simulink model "sampleModel1999"  (R2022a)
settings: Solver=FixedStepAuto  StartTime=0.0  StopTime=10.0  RelTol=1e-3
undefined symbols (not defined in the file): DiscIntNeverNeededParam, magnitude, Newton, Raphson
libraries: simulink x51, slpidlib x21
(part 1 of 3)
settings Model: SimulationMode=software-in-the-loop (sil)  Creator=lenovo  LastModifiedBy=TSMC
settings DataIOCC: InspectSignalLogs=on  SignalLoggingName=logsOut
settings OptimizationCC: DefaultParameterBehavior=Inlined  EnhancedBackFolding=on  PassReuseOutputArgsAs=Individual arguments  ZeroExternalMemoryAtStartup=off  ZeroInternalMemoryAtStartup=off  OptimizeBlockOrder=speed  DifferentSizesBufferReuse=on  OptimizationCustomize=off  EfficientTunableParamExpr=on
settings DebuggingCC: ParameterTunabilityLossMsg=error  UnconnectedInputMsg=warning  UnconnectedOutputMsg=warning  UnconnectedLineMsg=warning
settings ModelReferenceCC: UpdateModelReferenceTargets=Force
settings SFSimCC: MATLABDynamicMemAlloc=off
settings RTWCC: SystemTargetFile=ert.tlc  TemplateMakefile=ert_default_tmf  GenerateReport=on  IncludeHyperlinkInReport=on  GenerateTraceInfo=on  DLArmComputeVersion=19.05
settings CodeAppCC: ForceParamTrailComments=on  IgnoreCustomStorageClasses=off  OperatorAnnotations=on  SimulinkDataObjDesc=on  SFDataObjDesc=on  InsertBlockDesc=on
settings ERTTargetCC: TargetLangStandard=C99 (ISO)  GenerateSampleERTMain=on  SupportContinuousTime=on  InlinedParameterPlacement=NonHierarchical  ERTCustomFileTemplate=example_file_process.tlc

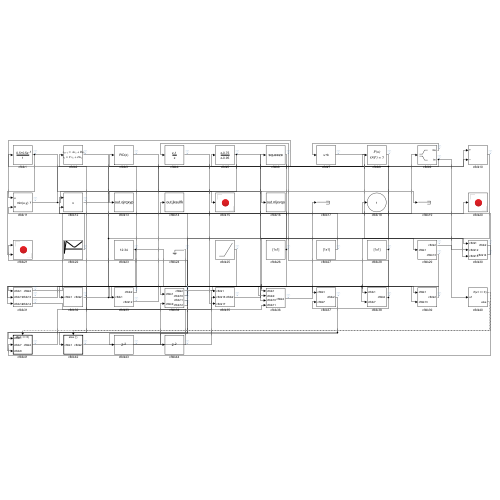
[thumbnail: Simulink's stored preview of the top-level diagram]
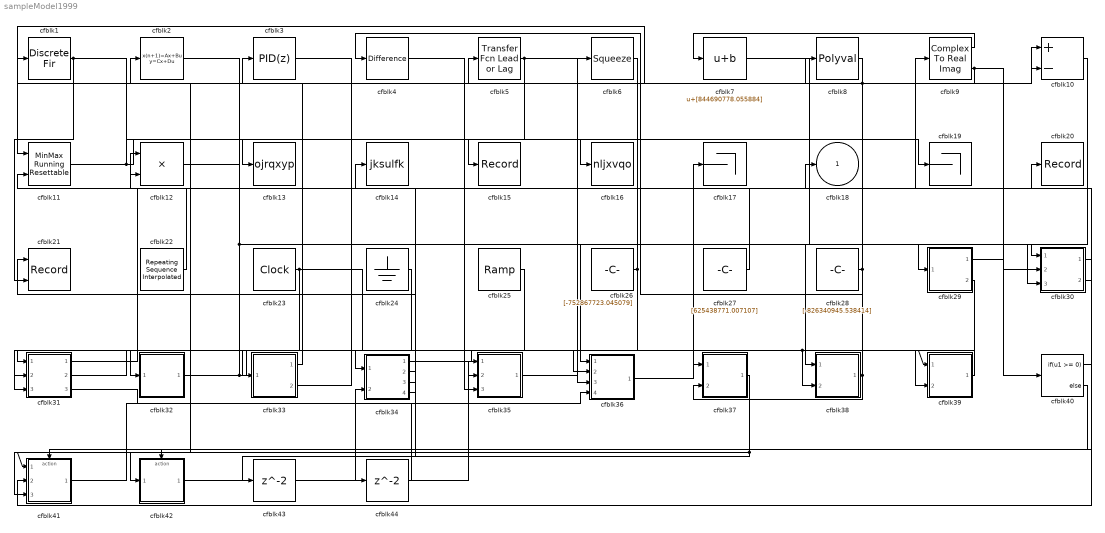
== system sampleModel1999 ==
  cfblk1 : DiscreteFir  SampleTime=1
  cfblk10 : Sum  Inputs=+-
  cfblk11 : simulink/Math Operations/MinMax Running Resettable  Function=min  vinit=0.0
  cfblk12 : Product  Inputs=**
  cfblk13 : ToWorkspace  VariableName=ojrqxyp  SaveFormat=Timeseries  SampleTime=-1
  cfblk14 : ToWorkspace  VariableName=jksulfk  SaveFormat=Timeseries  SampleTime=-1
  cfblk15 : Record  FileSettingsInternal="{\"entries\":[{\"content\":{\"excelSettings\":{\"content\":{},\"type\":\"Streamout.ExcelSettings\"}},\"type\":\"Streamout.FileSettingStorage\",\"uuid\":\"90b2dc24-f850-46d1-98e9-7d4ead9faf76\"}],\"packageUris\":[\"http://schema.mathworks.com/mf0/streamout_blocks/R2020a\"],\"version\":\"1.0\"}"  SignalsInternal="{\"entries\":[{\"content\":{\"signals\":[]},\"type\":\"RecordBlkView.InputSignals\",\"uuid\":\"4951badd-dc58-422e-9e9b-efd1dd601589\"}],\"packageUris\":[\"http://schema.mathworks.com/mf0/streamout_blocks/R2020a\"],\"version\":\"1.0\"}"  VisualizationBindings="{\"sparklinesplugin\":{\"info\":[{\"bindingParametersList\":[],\"subplotID\":1}]}}"
  cfblk16 : ToWorkspace  VariableName=nljxvqo  SaveFormat=Timeseries  SampleTime=-1
  cfblk17 : Terminator
  cfblk19 : Terminator
  cfblk2 : DiscreteStateSpace
  cfblk20 : Record  FileSettingsInternal="{\"entries\":[{\"content\":{\"excelSettings\":{\"content\":{},\"type\":\"Streamout.ExcelSettings\"}},\"type\":\"Streamout.FileSettingStorage\",\"uuid\":\"17e1182a-0793-4fff-8a02-480c6dfdb997\"}],\"packageUris\":[\"http://schema.mathworks.com/mf0/streamout_blocks/R2020a\"],\"version\":\"1.0\"}"  SignalsInternal="{\"entries\":[{\"content\":{\"signals\":[]},\"type\":\"RecordBlkView.InputSignals\",\"uuid\":\"65f435e3-1ce2-412d-96a0-f220de8eba44\"}],\"packageUris\":[\"http://schema.mathworks.com/mf0/streamout_blocks/R2020a\"],\"version\":\"1.0\"}"  VisualizationBindings="{\"sparklinesplugin\":{\"info\":[{\"bindingParametersList\":[],\"subplotID\":1}]}}"
  cfblk21 : Record  FileSettingsInternal="{\"entries\":[{\"content\":{\"excelSettings\":{\"content\":{},\"type\":\"Streamout.ExcelSettings\"}},\"type\":\"Streamout.FileSettingStorage\",\"uuid\":\"712499bb-47a7-4324-9665-446955fb75ef\"}],\"packageUris\":[\"http://schema.mathworks.com/mf0/streamout_blocks/R2020a\"],\"version\":\"1.0\"}"  Layout=[1 1]  SignalsInternal="{\"entries\":[{\"content\":{\"signals\":[]},\"type\":\"RecordBlkView.InputSignals\",\"uuid\":\"d2038af1-ceeb-4d6d-b80f-55793e10b03b\"}],\"packageUris\":[\"http://schema.mathworks.com/mf0/streamout_blocks/R2020a\"],\"version\":\"1.0\"}"  VisualizationBindings="{\"xyplotplugin\":{\"info\":[{\"series\":[],\"subplotID\":1}]}}"  CompatibilityTag=XY  st=-1
  cfblk22 : simulink/Sources/Repeating Sequence Interpolated  OutValues=[-485646331.647212, 895001609.068764, 235742497.742022, 228091536.709134, 839624606.118321]  TimeValues=[0 0.1 0.5 0.6 1].'  LookUpMeth=Use Input Below  tsamp=0.01  OutMin=[]  OutMax=[]  OutDataTypeStr=double  OutputDataTypeScalingMode=double  OutDataType=fixdt(0,8)  OutScaling=2^-10
  cfblk23 : DigitalClock
  cfblk24 : Ground
  cfblk25 : simulink/Sources/Ramp  slope=[-4406.456708]  start=[7.098891]  InitialOutput=[-211121.092474]
  cfblk26 : Constant  Value=[-752867723.045079]  SampleTime=1
  cfblk27 : Constant  Value=[625438771.007107]  SampleTime=1
  cfblk28 : Constant  Value=[-826340945.538414]  SampleTime=1
  cfblk29 : Subsystem
  cfblk3 : slpidlib/PID Controller  Controller=PID  Form=Parallel  TimeDomain=Discrete-time  UseExternalTs=off  SampleTime=1  IntegratorMethod=Forward Euler  FilterMethod=Forward Euler  ControllerParametersSource=internal  P=1  I=1  UseKiTs=off  D=0  N=100  UseFilter=on  TunerSelectOption=Transfer Function Based (PID Tuner App)  InitialConditionSource=internal  InitialConditionForIntegrator=0  InitialConditionForFilter=0  DifferentiatorICPrevScaledInput=0  ExternalReset=none  TrackingMode=off  Kt=1  LimitOutput=off  SatLimitsSource=internal  UpperSaturationLimit=inf  LowerSaturationLimit=-inf  LinearizeAsGain=off  AntiWindupMode=none  Kb=1  POutMin=[]  POutMax=[]  IOutMin=[]  IOutMax=[]  DOutMin=[]  DOutMax=[]  NOutMin=[]  NOutMax=[]  SumOutMin=[]  SumOutMax=[]  SaturationOutMin=[]  SaturationOutMax=[]  PParamMin=[]  PParamMax=[]  IParamMin=[]  IParamMax=[]  DParamMin=[]  DParamMax=[]  NParamMin=[]  NParamMax=[]  KbParamMin=[]  KbParamMax=[]  KtParamMin=[]  KtParamMax=[]  KbOutMin=[]  KbOutMax=[]  KtOutMin=[]  KtOutMax=[]  IntegratorOutMin=[]  IntegratorOutMax=[]  FilterOutMin=[]  FilterOutMax=[]  SumI1OutMin=[]  SumI1OutMax=[]  SumI2OutMin=[]  SumI2OutMax=[]  SumI3OutMin=[]  SumI3OutMax=[]  SumI4OutMin=[]  SumI4OutMax=[]  SumDOutMin=[]  SumDOutMax=[]  DifferentiatorOutMin=[]  DifferentiatorOutMax=[]  FilterDiffOutCoefMin=[]  FilterDiffOutCoefMax=[]  ReciprocalOutMin=[]  ReciprocalOutMax=[]  SumDenOutMin=[]  SumDenOutMax=[]  SumNumOutMin=[]  SumNumOutMax=[]  DivideOutMin=[]  DivideOutMax=[]  UdiffTsProdOutMin=[]  UdiffTsProdOutMax=[]  NTsProdOutMin=[]  NTsProdOutMax=[]  UintegralTsProdOutMin=[]  UintegralTsProdOutMax=[]  UngainTsProdOutMin=[]  UngainTsProdOutMax=[]  IntegratorContinuousStateAttributes=''  IntegratorStateMustResolveToSignalObject=off  IntegratorRTWStateStorageClass=Auto  FilterContinuousStateAttributes=''  FilterStateMustResolveToSignalObject=off  FilterRTWStateStorageClass=Auto  ParallelPVariant=InternalParameters  IdealPVariant=Disabled  IVariant=InternalParameters  DVariant=InternalParameters  IntegratorVariant=Discrete  SatVariant=Disabled  AWVariant=Passthrough  PCopyVariant=Disabled  TRVariant=Disabled  FdbkBlocksVariant=Forward  IdealPFdbkVariant=Disabled  SatFdbkVariant=Disabled  DerivativeFilterVariant=ForwardEulerFilter  NVariant=InternalParameters  NCopyVariant=Disabled  FilterICVariant=InternalICsFilter  IntegratorICVariant=InternalICs  ExternalResetVariant=Disabled  TRSumVariant=Passthrough  SumFdbkVariant=Disabled  SumVariant=Sum_PID  TsampFilterVariant=InternalTs  TsampNgainVariant=Passthrough  TsampIntegralVariant=Passthrough  ExternalSaturationOutDataTypeStr=Inherit: Same as second input  aMode=0
  cfblk30 : Subsystem
  cfblk31 : Subsystem
  cfblk32 : Subsystem
  cfblk33 : Subsystem
  cfblk34 : Subsystem
  cfblk35 : Subsystem
  cfblk36 : Subsystem
  cfblk37 : Subsystem
  cfblk38 : Subsystem
  cfblk39 : Subsystem
  cfblk4 : simulink/Discrete/Difference  ICPrevInput=0.0  OutMin=[]  OutMax=[]  OutDataTypeStr=Inherit: Inherit via back propagation  OutDataType=fixdt(1, 16)  OutScaling=2^-10  DoSatur=off
  cfblk40 : If  IfExpression=u1 >= 0  SampleTime=1
  cfblk41 : Subsystem  TreatAsAtomicUnit=on
  cfblk42 : Subsystem  TreatAsAtomicUnit=on
  cfblk43 : Delay  SampleTime=1
  cfblk44 : Delay  SampleTime=1
  cfblk5 : simulink/Discrete/Transfer Fcn Lead or Lag  PoleZ=0.95  ZeroZ=0.75  ICPrevOutput=0.0  ICPrevInput=0.0  DoSatur=off
      settings: SourceProductBaseCode=SL
  cfblk6 : Squeeze
  cfblk7 : Bias  Bias=[844690778.055884]  SaturateOnIntegerOverflow=off
  cfblk8 : Polyval  Coefs=[ +2.081618890e-019, -1.441693666e-014, +4.719686976e-010, -8.536869453e-006, +1.621573104e-001, -8.087801117e+001 ]
  cfblk9 : ComplexToRealImag
  cfblk18 : Outport
  wires:
  cfblk37/1(cfblk2) -> cfblk41/1(cfblk1), cfblk43/1
  cfblk6/1 -> cfblk36/1(cfblk1)
  cfblk38/1(cfblk2) -> cfblk4/1, cfblk37/2(cfblk7)
  cfblk9/1 -> cfblk7/1
  cfblk32/1(cfblk2) -> cfblk36/2(cfblk9), cfblk20/1
  cfblk8/1 -> cfblk11/1, cfblk38/1(cfblk1)
  cfblk28/1 -> cfblk1/1, cfblk31/3(cfblk12)
  cfblk3/1 -> cfblk16/1
  cfblk5/1 -> cfblk13/1, cfblk30/1(cfblk1)
  cfblk36/1(cfblk2) -> cfblk17/1
  cfblk9/2 -> cfblk5/1, cfblk30/2(cfblk12)
  cfblk33/1(cfblk2) -> cfblk3/1
  cfblk11/1 -> cfblk19/1, cfblk10/2
  cfblk7/1 -> cfblk29/1(cfblk1)
  cfblk4/1 -> cfblk36/3(cfblk10)
  cfblk1/1 -> cfblk15/1, cfblk21/2
  cfblk31/1(cfblk2) -> cfblk9/1
  cfblk30/1(cfblk2) -> cfblk41/2(cfblk7)
  cfblk25/1 -> cfblk32/1(cfblk1)
  cfblk26/1 -> cfblk12/1, cfblk31/2(cfblk11)
  cfblk22/1 -> cfblk11/2
  cfblk24/1 -> cfblk42/1(cfblk1)
  cfblk41/1(cfblk2) -> cfblk36/4(cfblk11)
  cfblk34/1(cfblk2) -> cfblk37/1(cfblk1)
  cfblk34/2(cfblk10) -> cfblk12/2
  cfblk12/1 -> cfblk10/1
  cfblk27/1 -> cfblk14/1
  cfblk2/1 -> cfblk39/1(cfblk1), cfblk38/2(cfblk7), cfblk30/3(cfblk13)
  cfblk34/3(cfblk11) -> cfblk41/3(cfblk8)
  cfblk34/4(cfblk12) -> cfblk21/1
  cfblk31/2(cfblk13) -> cfblk34/1(cfblk1)
  cfblk35/1(cfblk2) -> cfblk6/1
  cfblk42/1(cfblk2) -> cfblk35/1(cfblk1)
  cfblk30/2(cfblk14) -> cfblk18/1
  cfblk23/1 -> cfblk33/1(cfblk1), cfblk39/2(cfblk13)
  cfblk29/1(cfblk2) -> cfblk40/1
  cfblk33/2(cfblk12) -> cfblk8/1
  cfblk31/3(cfblk14) -> cfblk35/2(cfblk16)
  cfblk39/1(cfblk2) -> cfblk31/1(cfblk1)
  cfblk29/2(cfblk13) -> cfblk35/3(cfblk17)
  cfblk40/1 -> cfblk41/Action
  cfblk40/2 -> cfblk42/Action
  cfblk43/1 -> cfblk34/2(cfblk9)
  cfblk10/1 -> cfblk44/1
  cfblk44/1 -> cfblk2/1

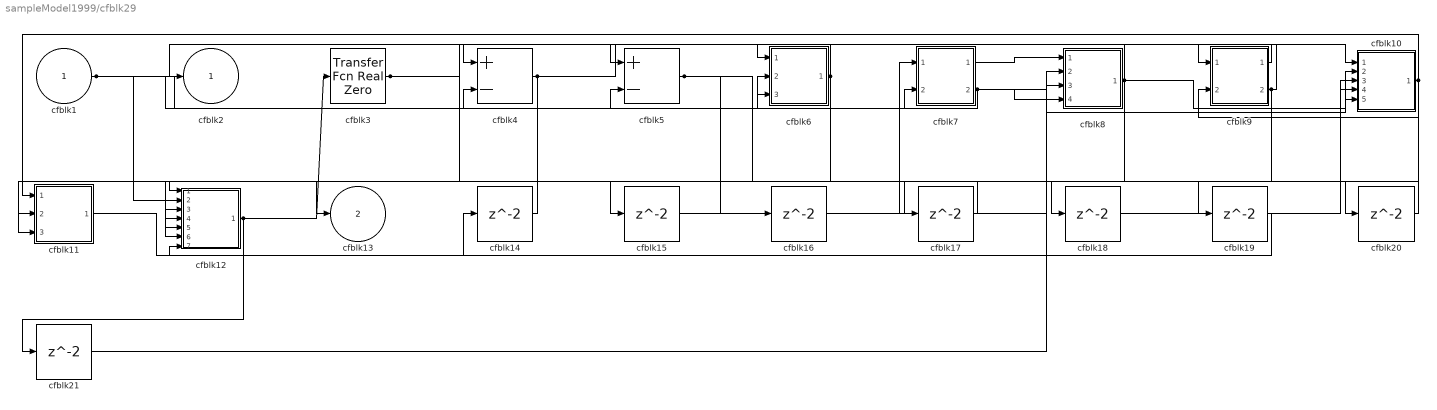
== system sampleModel1999/cfblk29 ==
  cfblk1 : Inport
  cfblk10 : Subsystem
  cfblk11 : Subsystem
  cfblk12 : Subsystem
  cfblk{14..21} (8 alike) : Delay  SampleTime=1
  cfblk3 : simulink/Discrete/Transfer Fcn Real Zero  ZeroZ=0.75  ICPrevInput=0.0  DoSatur=off
      settings: SourceProductBaseCode=SL
  cfblk4 : Sum  Inputs=+-
  cfblk5 : Sum  Inputs=+-
  cfblk6 : Subsystem
  cfblk7 : Subsystem
  cfblk8 : Subsystem
  cfblk9 : Subsystem
  cfblk2 : Outport
  cfblk13 : Outport  Port=2
  wires:
  cfblk7/1(cfblk2) -> cfblk8/1(cfblk1)
  cfblk9/1(cfblk2) -> cfblk6/1(cfblk1)
  cfblk5/1 -> cfblk16/1, cfblk17/1, cfblk18/1
  cfblk1/1 -> cfblk7/2(cfblk13), cfblk5/2, cfblk12/2(cfblk11)
  cfblk8/1(cfblk2) -> cfblk4/1, cfblk12/1(cfblk1), cfblk10/5(cfblk13)
  cfblk4/1 -> cfblk10/1(cfblk1), cfblk13/1, cfblk12/5(cfblk14), cfblk12/6(cfblk15)
  cfblk9/2(cfblk8) -> cfblk5/1, cfblk11/3(cfblk11), cfblk19/1
  cfblk12/1(cfblk2) -> cfblk3/1, cfblk21/1
  cfblk7/2(cfblk14) -> cfblk6/2(cfblk10), cfblk6/3(cfblk11), cfblk10/2(cfblk10), cfblk8/4(cfblk12)
  cfblk6/1(cfblk2) -> cfblk2/1, cfblk15/1
  cfblk3/1 -> cfblk9/1(cfblk1), cfblk20/1
  cfblk10/1(cfblk2) -> cfblk11/1(cfblk1), cfblk11/2(cfblk10), cfblk12/4(cfblk13), cfblk9/2(cfblk7)
  cfblk11/1(cfblk2) -> cfblk14/1
  cfblk14/1 -> cfblk4/2
  cfblk15/1 -> cfblk8/2(cfblk10)
  cfblk16/1 -> cfblk7/1(cfblk1)
  cfblk17/1 -> cfblk12/3(cfblk12)
  cfblk18/1 -> cfblk10/4(cfblk12)
  cfblk19/1 -> cfblk12/7(cfblk16)
  cfblk20/1 -> cfblk10/3(cfblk11)
  cfblk21/1 -> cfblk8/3(cfblk11)

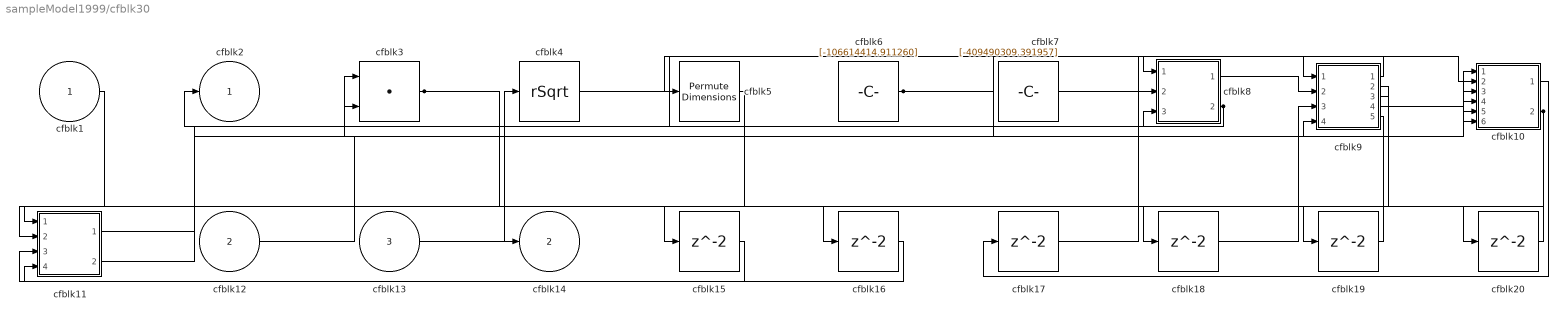
== system sampleModel1999/cfblk30 ==
  cfblk1 : Inport
  cfblk12 : Inport  Port=2
  cfblk13 : Inport  Port=3
  cfblk10 : Subsystem
  cfblk11 : Subsystem
  cfblk{15..20} (6 alike) : Delay  SampleTime=1
  cfblk3 : DotProduct  OutDataTypeStr=Inherit: Inherit via internal rule
  cfblk4 : Sqrt  Operator=rSqrt  AlgorithmType=Newton-Raphson
  cfblk5 : PermuteDimensions
  cfblk6 : Constant  Value=[-106614414.911260]  SampleTime=1
  cfblk7 : Constant  Value=[-409490309.391957]  SampleTime=1
  cfblk8 : Subsystem
  cfblk9 : Subsystem
  cfblk2 : Outport
  cfblk14 : Outport  Port=2
  wires:
  cfblk1/1 -> cfblk11/1(cfblk1)
  cfblk3/1 -> cfblk10/5(cfblk15), cfblk20/1
  cfblk11/1(cfblk2) -> cfblk8/1(cfblk1)
  cfblk12/1 -> cfblk10/1(cfblk1)
  cfblk13/1 -> cfblk4/1
  cfblk4/1 -> cfblk8/3(cfblk10)
  cfblk6/1 -> cfblk10/2(cfblk12), cfblk10/6(cfblk16)
  cfblk9/1(cfblk2) -> cfblk5/1
  cfblk7/1 -> cfblk9/1(cfblk1)
  cfblk8/1(cfblk2) -> cfblk9/2(cfblk7)
  cfblk9/2(cfblk10) -> cfblk14/1
  cfblk8/2(cfblk11) -> cfblk2/1, cfblk3/2
  cfblk9/4(cfblk12) -> cfblk10/3(cfblk13)
  cfblk11/2(cfblk15) -> cfblk10/4(cfblk14)
  cfblk10/2(cfblk17) -> cfblk18/1, cfblk19/1
  cfblk9/5(cfblk13) -> cfblk3/1
  cfblk5/1 -> cfblk15/1
  cfblk15/1 -> cfblk11/3(cfblk13)
  cfblk9/3(cfblk11) -> cfblk16/1
  cfblk16/1 -> cfblk11/4(cfblk14)
  cfblk10/1(cfblk2) -> cfblk17/1
  cfblk17/1 -> cfblk8/2(cfblk9)
  cfblk18/1 -> cfblk9/3(cfblk8)
  cfblk19/1 -> cfblk9/4(cfblk9)
  cfblk20/1 -> cfblk11/2(cfblk12)

== system sampleModel1999/cfblk31 ==
  cfblk1 : Inport
  cfblk11 : Inport  Port=2
  cfblk12 : Inport  Port=3
  cfblk10 : Subsystem
  cfblk15 : Delay  SampleTime=1
  cfblk16 : Delay  SampleTime=1
  cfblk3 : DiscreteZeroPole  Poles=[0 0.5]  Gain=1
  cfblk4 : slpidlib/PID Controller  Controller=PID  Form=Parallel  TimeDomain=Discrete-time  UseExternalTs=off  SampleTime=1  IntegratorMethod=Forward Euler  FilterMethod=Forward Euler  ControllerParametersSource=internal  P=1  I=1  UseKiTs=off  D=0  N=100  UseFilter=on  TunerSelectOption=Transfer Function Based (PID Tuner App)  InitialConditionSource=internal  InitialConditionForIntegrator=0  InitialConditionForFilter=0  DifferentiatorICPrevScaledInput=0  ExternalReset=none  TrackingMode=off  Kt=1  LimitOutput=off  SatLimitsSource=internal  UpperSaturationLimit=inf  LowerSaturationLimit=-inf  LinearizeAsGain=off  AntiWindupMode=none  Kb=1  POutMin=[]  POutMax=[]  IOutMin=[]  IOutMax=[]  DOutMin=[]  DOutMax=[]  NOutMin=[]  NOutMax=[]  SumOutMin=[]  SumOutMax=[]  SaturationOutMin=[]  SaturationOutMax=[]  PParamMin=[]  PParamMax=[]  IParamMin=[]  IParamMax=[]  DParamMin=[]  DParamMax=[]  NParamMin=[]  NParamMax=[]  KbParamMin=[]  KbParamMax=[]  KtParamMin=[]  KtParamMax=[]  KbOutMin=[]  KbOutMax=[]  KtOutMin=[]  KtOutMax=[]  IntegratorOutMin=[]  IntegratorOutMax=[]  FilterOutMin=[]  FilterOutMax=[]  SumI1OutMin=[]  SumI1OutMax=[]  SumI2OutMin=[]  SumI2OutMax=[]  SumI3OutMin=[]  SumI3OutMax=[]  SumI4OutMin=[]  SumI4OutMax=[]  SumDOutMin=[]  SumDOutMax=[]  DifferentiatorOutMin=[]  DifferentiatorOutMax=[]  FilterDiffOutCoefMin=[]  FilterDiffOutCoefMax=[]  ReciprocalOutMin=[]  ReciprocalOutMax=[]  SumDenOutMin=[]  SumDenOutMax=[]  SumNumOutMin=[]  SumNumOutMax=[]  DivideOutMin=[]  DivideOutMax=[]  UdiffTsProdOutMin=[]  UdiffTsProdOutMax=[]  NTsProdOutMin=[]  NTsProdOutMax=[]  UintegralTsProdOutMin=[]  UintegralTsProdOutMax=[]  UngainTsProdOutMin=[]  UngainTsProdOutMax=[]  IntegratorContinuousStateAttributes=''  IntegratorStateMustResolveToSignalObject=off  IntegratorRTWStateStorageClass=Auto  FilterContinuousStateAttributes=''  FilterStateMustResolveToSignalObject=off  FilterRTWStateStorageClass=Auto  ParallelPVariant=InternalParameters  IdealPVariant=Disabled  IVariant=InternalParameters  DVariant=InternalParameters  IntegratorVariant=Discrete  SatVariant=Disabled  AWVariant=Passthrough  PCopyVariant=Disabled  TRVariant=Disabled  FdbkBlocksVariant=Forward  IdealPFdbkVariant=Disabled  SatFdbkVariant=Disabled  DerivativeFilterVariant=ForwardEulerFilter  NVariant=InternalParameters  NCopyVariant=Disabled  FilterICVariant=InternalICsFilter  IntegratorICVariant=InternalICs  ExternalResetVariant=Disabled  TRSumVariant=Passthrough  SumFdbkVariant=Disabled  SumVariant=Sum_PID  TsampFilterVariant=InternalTs  TsampNgainVariant=Passthrough  TsampIntegralVariant=Passthrough  ExternalSaturationOutDataTypeStr=Inherit: Same as second input  aMode=0
  cfblk5 : Abs  SaturateOnIntegerOverflow=off
  cfblk6 : Constant  Value=[386910911.737461]  SampleTime=1
  cfblk7 : Subsystem
  cfblk8 : Subsystem
  cfblk9 : Subsystem
  cfblk2 : Outport
  cfblk13 : Outport  Port=2
  cfblk14 : Outport  Port=3
  wires:
  cfblk3/1 -> cfblk2/1
  cfblk6/1 -> cfblk8/2(cfblk8), cfblk9/4(cfblk9)
  cfblk10/1(cfblk2) -> cfblk3/1
  cfblk12/1 -> cfblk13/1
  cfblk9/1(cfblk2) -> cfblk7/1(cfblk1)
  cfblk10/2(cfblk15) -> cfblk7/2(cfblk8)
  cfblk4/1 -> cfblk10/1(cfblk1), cfblk9/2(cfblk7), cfblk9/5(cfblk10)
  cfblk1/1 -> cfblk8/3(cfblk9)
  cfblk8/1(cfblk2) -> cfblk5/1
  cfblk11/1 -> cfblk10/2(cfblk14), cfblk9/3(cfblk8), cfblk7/3(cfblk9), cfblk7/4(cfblk10)
  cfblk5/1 -> cfblk9/1(cfblk1)
  cfblk7/2(cfblk11) -> cfblk14/1
  cfblk7/1(cfblk2) -> cfblk15/1
  cfblk15/1 -> cfblk8/1(cfblk1)
  cfblk10/3(cfblk16) -> cfblk16/1
  cfblk16/1 -> cfblk4/1

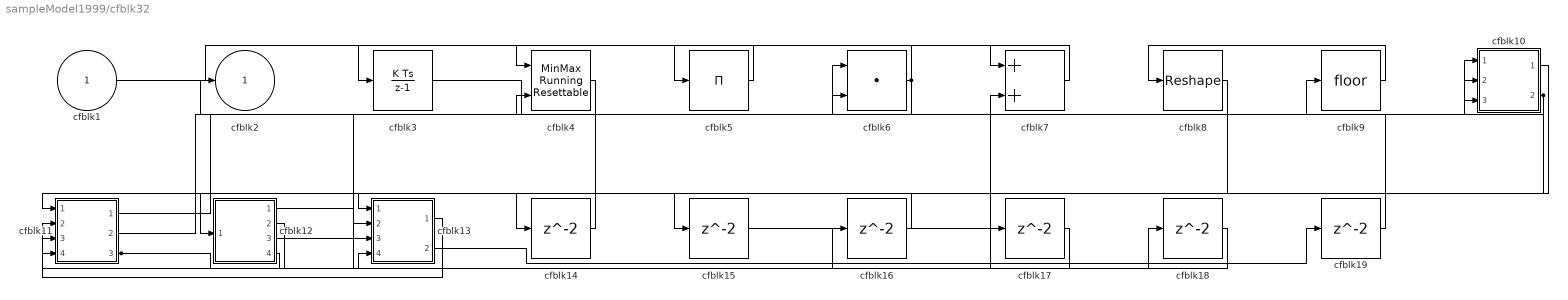
== system sampleModel1999/cfblk32 ==
  cfblk1 : Inport
  cfblk10 : Subsystem
  cfblk11 : Subsystem
  cfblk12 : Subsystem
  cfblk13 : Subsystem
  cfblk{14..19} (6 alike) : Delay  SampleTime=1
  cfblk3 : DiscreteIntegrator  ICPrevOutput=DiscIntNeverNeededParam  ICPrevScaledInput=DiscIntNeverNeededParam
  cfblk4 : simulink/Math Operations/MinMax Running Resettable  Function=min  vinit=0.0
  cfblk5 : Product  Inputs=*
  cfblk6 : DotProduct  OutDataTypeStr=Inherit: Inherit via internal rule
  cfblk7 : Sum
  cfblk8 : Reshape
  cfblk9 : Rounding
  cfblk2 : Outport
  wires:
  cfblk11/1(cfblk2) -> cfblk10/1(cfblk1)
  cfblk8/1 -> cfblk12/1(cfblk1)
  cfblk7/1 -> cfblk5/1
  cfblk5/1 -> cfblk3/1
  cfblk9/1 -> cfblk8/1
  cfblk1/1 -> cfblk7/1
  cfblk4/1 -> cfblk13/1(cfblk1)
  cfblk6/1 -> cfblk4/1, cfblk4/2
  cfblk12/1(cfblk2) -> cfblk6/1
  cfblk10/2(cfblk12) -> cfblk2/1, cfblk15/1
  cfblk11/2(cfblk12) -> cfblk10/2(cfblk10)
  cfblk11/3(cfblk13) -> cfblk16/1, cfblk17/1, cfblk18/1
  cfblk13/1(cfblk2) -> cfblk11/2(cfblk9)
  cfblk12/2(cfblk13) -> cfblk11/3(cfblk10)
  cfblk3/1 -> cfblk9/1
  cfblk12/3(cfblk14) -> cfblk10/3(cfblk11)
  cfblk12/4(cfblk15) -> cfblk11/4(cfblk11)
  cfblk10/1(cfblk2) -> cfblk14/1
  cfblk14/1 -> cfblk11/1(cfblk1)
  cfblk15/1 -> cfblk7/2
  cfblk16/1 -> cfblk13/2(cfblk8)
  cfblk17/1 -> cfblk13/3(cfblk9)
  cfblk18/1 -> cfblk13/4(cfblk10)
  cfblk13/2(cfblk11) -> cfblk19/1
  cfblk19/1 -> cfblk6/2

== system sampleModel1999/cfblk33 ==
  cfblk1 : Inport
  cfblk10 : Subsystem
  cfblk11 : Subsystem
  cfblk13 : Delay  SampleTime=1
  cfblk14 : Delay  SampleTime=1
  cfblk3 : DiscreteTransferFcn  SampleTime=1
  cfblk4 : PermuteDimensions
  cfblk5 : Product  Inputs=*
  cfblk6 : Abs  SaturateOnIntegerOverflow=off
  cfblk7 : Constant  Value=[-887141361.180652]  SampleTime=1
  cfblk8 : Subsystem
  cfblk9 : Subsystem
  cfblk2 : Outport
  cfblk12 : Outport  Port=2
  wires:
  cfblk3/1 -> cfblk5/1, cfblk10/3(cfblk14), cfblk10/4(cfblk15)
  cfblk7/1 -> cfblk2/1
  cfblk4/1 -> cfblk3/1, cfblk12/1
  cfblk1/1 -> cfblk11/1(cfblk1), cfblk11/2(cfblk12)
  cfblk5/1 -> cfblk8/2(cfblk14)
  cfblk6/1 -> cfblk8/3(cfblk15), cfblk10/2(cfblk13)
  cfblk9/1(cfblk2) -> cfblk4/1
  cfblk8/1(cfblk2) -> cfblk10/1(cfblk1)
  cfblk11/1(cfblk2) -> cfblk9/1(cfblk1)
  cfblk9/2(cfblk17) -> cfblk6/1
  cfblk10/1(cfblk2) -> cfblk13/1
  cfblk13/1 -> cfblk8/1(cfblk1)
  cfblk8/2(cfblk16) -> cfblk14/1
  cfblk14/1 -> cfblk9/2(cfblk16)

== system sampleModel1999/cfblk34 ==
  cfblk1 : Inport
  cfblk9 : Inport  Port=2
  cfblk3 : Bias  Bias=[203948966.941377]  SaturateOnIntegerOverflow=off
  cfblk4 : Trigonometry
  cfblk5 : Sqrt
  cfblk6 : Assignment  DiagnosticForDimensions=Warning  IndexOptions=Index vector (dialog)  Indices=1  OutputSizes=1
  cfblk7 : Subsystem
  cfblk8 : Subsystem
  cfblk2 : Outport
  cfblk10 : Outport  Port=2
  cfblk11 : Outport  Port=3
  cfblk12 : Outport  Port=4
  wires:
  cfblk9/1 -> cfblk6/1
  cfblk5/1 -> cfblk4/1
  cfblk7/1(cfblk2) -> cfblk6/2
  cfblk7/2(cfblk9) -> cfblk3/1
  cfblk3/1 -> cfblk10/1, cfblk5/1
  cfblk8/1(cfblk2) -> cfblk12/1
  cfblk1/1 -> cfblk7/1(cfblk1), cfblk8/2(cfblk7), cfblk7/2(cfblk7), cfblk7/3(cfblk8)
  cfblk4/1 -> cfblk8/1(cfblk1)
  cfblk6/1 -> cfblk2/1
  cfblk8/2(cfblk8) -> cfblk11/1

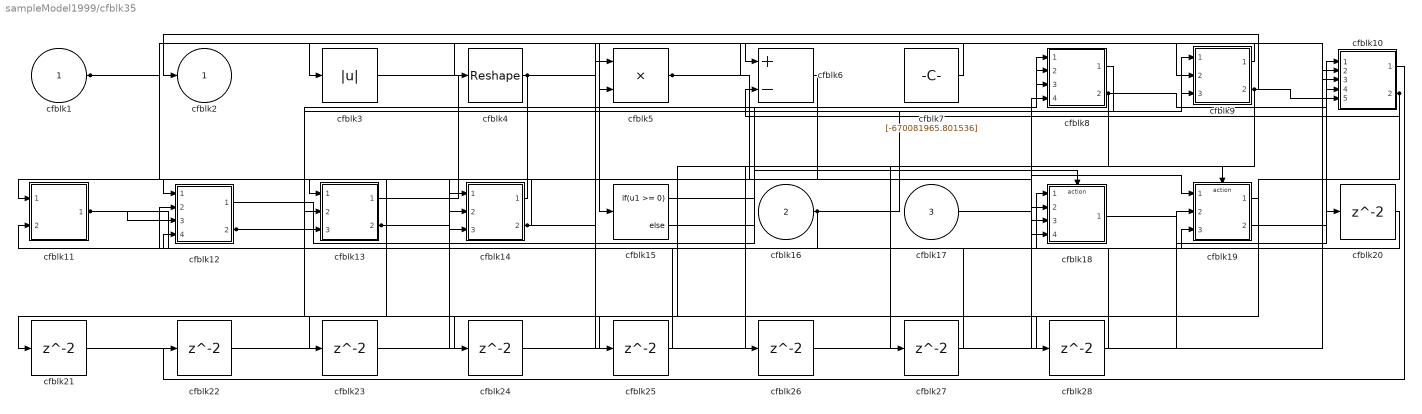
== system sampleModel1999/cfblk35 ==
  cfblk1 : Inport
  cfblk16 : Inport  Port=2
  cfblk17 : Inport  Port=3
  cfblk10 : Subsystem
  cfblk11 : Subsystem
  cfblk12 : Subsystem
  cfblk13 : Subsystem
  cfblk14 : Subsystem
  cfblk15 : If  IfExpression=u1 >= 0  SampleTime=1
  cfblk18 : Subsystem  TreatAsAtomicUnit=on
  cfblk19 : Subsystem  TreatAsAtomicUnit=on
  cfblk{20..28} (9 alike) : Delay  SampleTime=1
  cfblk3 : Abs  SaturateOnIntegerOverflow=off
  cfblk4 : Reshape
  cfblk5 : Product  Inputs=**
  cfblk6 : Sum  Inputs=+-
  cfblk7 : Constant  Value=[-670081965.801536]  SampleTime=1
  cfblk8 : Subsystem
  cfblk9 : Subsystem
  cfblk2 : Outport
  wires:
  cfblk16/1 -> cfblk9/1(cfblk1), cfblk11/2(cfblk13)
  cfblk9/1(cfblk2) -> cfblk15/1
  cfblk9/2(cfblk17) -> cfblk2/1, cfblk10/5(cfblk14), cfblk25/1, cfblk26/1
  cfblk12/1(cfblk2) -> cfblk8/1(cfblk1)
  cfblk11/1(cfblk2) -> cfblk18/1(cfblk1), cfblk12/3(cfblk15)
  cfblk5/1 -> cfblk18/2(cfblk15), cfblk9/2(cfblk15)
  cfblk13/1(cfblk2) -> cfblk18/3(cfblk16)
  cfblk3/1 -> cfblk18/4(cfblk17)
  cfblk14/1(cfblk2) -> cfblk13/1(cfblk1)
  cfblk12/2(cfblk17) -> cfblk9/3(cfblk16), cfblk8/3(cfblk12), cfblk28/1
  cfblk4/1 -> cfblk6/1, cfblk13/3(cfblk11)
  cfblk10/2(cfblk15) -> cfblk6/2, cfblk24/1
  cfblk1/1 -> cfblk14/3(cfblk15), cfblk3/1, cfblk10/3(cfblk12)
  cfblk13/2(cfblk12) -> cfblk12/1(cfblk1), cfblk19/3(cfblk12)
  cfblk17/1 -> cfblk19/1(cfblk1)
  cfblk7/1 -> cfblk4/1
  cfblk14/2(cfblk16) -> cfblk11/1(cfblk1), cfblk8/2(cfblk11)
  cfblk19/2(cfblk13) -> cfblk10/1(cfblk1)
  cfblk8/1(cfblk2) -> cfblk5/2
  cfblk8/2(cfblk14) -> cfblk10/4(cfblk13), cfblk27/1
  cfblk15/1 -> cfblk18/Action
  cfblk15/2 -> cfblk19/Action
  cfblk18/1(cfblk2) -> cfblk20/1
  cfblk20/1 -> cfblk13/2(cfblk10)
  cfblk19/1(cfblk2) -> cfblk21/1
  cfblk21/1 -> cfblk14/1(cfblk1)
  cfblk10/1(cfblk2) -> cfblk22/1
  cfblk22/1 -> cfblk5/1
  cfblk6/1 -> cfblk23/1
  cfblk23/1 -> cfblk10/2(cfblk11)
  cfblk24/1 -> cfblk19/2(cfblk11)
  cfblk25/1 -> cfblk12/4(cfblk16)
  cfblk26/1 -> cfblk8/4(cfblk13)
  cfblk27/1 -> cfblk12/2(cfblk14)
  cfblk28/1 -> cfblk14/2(cfblk14)

== system sampleModel1999/cfblk36 ==
  cfblk1 : Inport
  cfblk9 : Inport  Port=2
  cfblk10 : Inport  Port=3
  cfblk11 : Inport  Port=4
  cfblk{12..15} (4 alike) : Delay  SampleTime=1
  cfblk3 : DiscreteIntegrator  ICPrevOutput=DiscIntNeverNeededParam  ICPrevScaledInput=DiscIntNeverNeededParam
  cfblk4 : Sum  Inputs=+
  cfblk5 : Math  Operator=pow
  cfblk6 : Subsystem
  cfblk7 : Subsystem
  cfblk8 : Subsystem
  cfblk2 : Outport
  wires:
  cfblk3/1 -> cfblk6/1(cfblk1), cfblk8/4(cfblk7)
  cfblk11/1 -> cfblk4/1
  cfblk10/1 -> cfblk6/2(cfblk12), cfblk8/5(cfblk8), cfblk7/5(cfblk12)
  cfblk5/1 -> cfblk13/1, cfblk14/1, cfblk15/1
  cfblk7/1(cfblk2) -> cfblk6/4(cfblk14)
  cfblk7/2(cfblk14) -> cfblk8/1(cfblk1)
  cfblk9/1 -> cfblk7/1(cfblk1)
  cfblk1/1 -> cfblk7/3(cfblk10), cfblk6/5(cfblk15)
  cfblk4/1 -> cfblk3/1, cfblk7/4(cfblk11), cfblk5/2
  cfblk8/2(cfblk9) -> cfblk5/1
  cfblk6/1(cfblk2) -> cfblk8/2(cfblk5)
  cfblk6/2(cfblk16) -> cfblk2/1
  cfblk8/1(cfblk2) -> cfblk12/1
  cfblk12/1 -> cfblk7/2(cfblk9)
  cfblk13/1 -> cfblk6/3(cfblk13)
  cfblk14/1 -> cfblk8/3(cfblk6)
  cfblk15/1 -> cfblk7/6(cfblk13)

== system sampleModel1999/cfblk37 ==
  cfblk1 : Inport
  cfblk7 : Inport  Port=2
  cfblk10 : Delay  SampleTime=1
  cfblk3 : Sum  Inputs=+
  cfblk4 : simulink/Math Operations/MinMax Running Resettable  Function=min  vinit=0.0
  cfblk5 : ComplexToRealImag
  cfblk6 : If  IfExpression=u1 >= 0  SampleTime=1
  cfblk8 : Subsystem  TreatAsAtomicUnit=on
  cfblk9 : Subsystem  TreatAsAtomicUnit=on
  cfblk2 : Outport
  wires:
  cfblk1/1 -> cfblk2/1, cfblk4/2
  cfblk7/1 -> cfblk3/1, cfblk8/4(cfblk8)
  cfblk4/1 -> cfblk9/1(cfblk1), cfblk6/1, cfblk5/1
  cfblk9/1(cfblk2) -> cfblk8/1(cfblk1), cfblk8/5(cfblk9)
  cfblk3/1 -> cfblk9/2(cfblk13), cfblk9/4(cfblk15)
  cfblk5/1 -> cfblk8/2(cfblk6)
  cfblk5/2 -> cfblk9/3(cfblk14), cfblk8/3(cfblk7)
  cfblk6/1 -> cfblk8/Action
  cfblk6/2 -> cfblk9/Action
  cfblk8/1(cfblk2) -> cfblk10/1
  cfblk10/1 -> cfblk4/1

== system sampleModel1999/cfblk38 ==
  cfblk1 : Inport
  cfblk7 : Inport  Port=2
  cfblk3 : Sqrt  Operator=rSqrt  AlgorithmType=Newton-Raphson
  cfblk4 : ComplexToRealImag
  cfblk5 : Subsystem
  cfblk6 : Subsystem
  cfblk8 : Delay  SampleTime=1
  cfblk2 : Outport
  wires:
  cfblk1/1 -> cfblk6/2(cfblk9)
  cfblk6/1(cfblk2) -> cfblk4/1, cfblk5/2(cfblk10)
  cfblk3/1 -> cfblk6/3(cfblk10)
  cfblk7/1 -> cfblk3/1
  cfblk4/1 -> cfblk2/1
  cfblk4/2 -> cfblk5/1(cfblk1)
  cfblk5/1(cfblk2) -> cfblk8/1
  cfblk8/1 -> cfblk6/1(cfblk1)

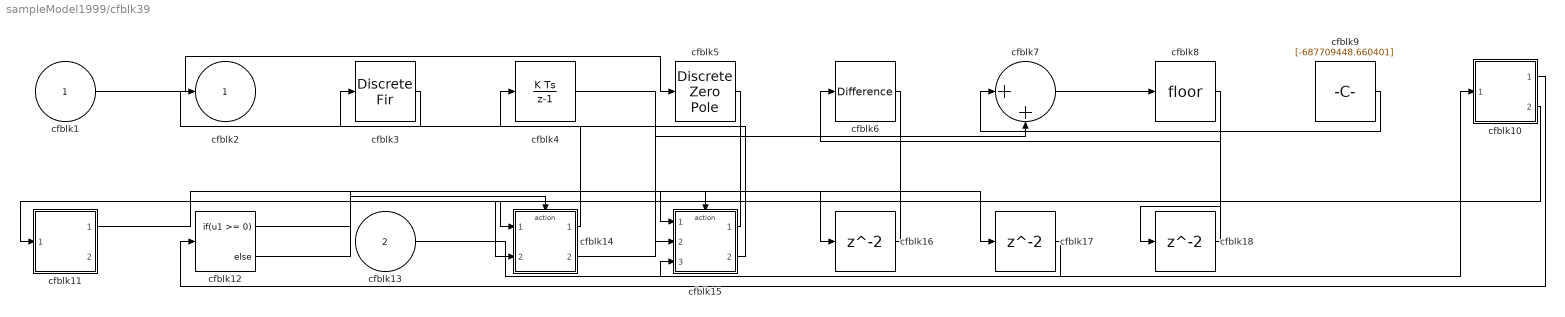
== system sampleModel1999/cfblk39 ==
  cfblk1 : Inport
  cfblk13 : Inport  Port=2
  cfblk10 : Subsystem
  cfblk11 : Subsystem
  cfblk12 : If  IfExpression=u1 >= 0  SampleTime=1
  cfblk14 : Subsystem  TreatAsAtomicUnit=on
  cfblk15 : Subsystem  TreatAsAtomicUnit=on
  cfblk16 : Delay  SampleTime=1
  cfblk17 : Delay  SampleTime=1
  cfblk18 : Delay  SampleTime=1
  cfblk3 : DiscreteFir  SampleTime=1
  cfblk4 : DiscreteIntegrator  ICPrevOutput=DiscIntNeverNeededParam  ICPrevScaledInput=DiscIntNeverNeededParam
  cfblk5 : DiscreteZeroPole  Poles=[0 0.5]  Gain=1
  cfblk6 : simulink/Discrete/Difference  ICPrevInput=0.0  OutMin=[]  OutMax=[]  OutDataTypeStr=Inherit: Inherit via back propagation  OutDataType=fixdt(1, 16)  OutScaling=2^-10  DoSatur=off
  cfblk7 : Sum  Inputs=|++
  cfblk8 : Rounding
  cfblk9 : Constant  Value=[-687709448.660401]  SampleTime=1
  cfblk2 : Outport
  wires:
  cfblk15/1(cfblk2) -> cfblk11/1(cfblk1)
  cfblk13/1 -> cfblk10/1(cfblk1)
  cfblk7/1 -> cfblk8/1
  cfblk1/1 -> cfblk5/1
  cfblk3/1 -> cfblk2/1
  cfblk5/1 -> cfblk15/2(cfblk12)
  cfblk10/1(cfblk2) -> cfblk12/1
  cfblk6/1 -> cfblk14/1(cfblk1)
  cfblk9/1 -> cfblk7/1
  cfblk15/2(cfblk14) -> cfblk4/1
  cfblk10/2(cfblk8) -> cfblk14/2(cfblk7)
  cfblk14/1(cfblk2) -> cfblk3/1
  cfblk14/2(cfblk8) -> cfblk7/2
  cfblk12/1 -> cfblk14/Action
  cfblk12/2 -> cfblk15/Action
  cfblk11/1(cfblk2) -> cfblk16/1
  cfblk16/1 -> cfblk15/1(cfblk1)
  cfblk4/1 -> cfblk17/1
  cfblk17/1 -> cfblk15/3(cfblk13)
  cfblk8/1 -> cfblk18/1
  cfblk18/1 -> cfblk6/1

== system sampleModel1999/cfblk41 ==
  cfblk1 : Inport
  cfblk7 : Inport  Port=2
  cfblk8 : Inport  Port=3
  Action Port : ActionPort  ActionPortLabel=if(u1 >= 0)
  cfblk3 : simulink/Discrete/Transfer Fcn Real Zero  ZeroZ=0.75  ICPrevInput=0.0  DoSatur=off
      settings: SourceProductBaseCode=SL
  cfblk4 : Sum  Inputs=|++
  cfblk5 : Trigonometry
  cfblk6 : Subsystem
  cfblk9 : Delay
  cfblk2 : Outport
  wires:
  cfblk8/1 -> cfblk6/1(cfblk1), cfblk6/4(cfblk7)
  cfblk5/1 -> cfblk4/1, cfblk6/3(cfblk6)
  cfblk3/1 -> cfblk5/1
  cfblk7/1 -> cfblk2/1
  cfblk1/1 -> cfblk3/1
  cfblk4/1 -> cfblk6/2(cfblk5)
  cfblk6/1(cfblk2) -> cfblk9/1
  cfblk9/1 -> cfblk4/2

== system sampleModel1999/cfblk42 ==
  cfblk1 : Inport
  Action Port : ActionPort  ActionPortLabel=else
  cfblk3 : slpidlib/PID Controller  Controller=PID  Form=Parallel  TimeDomain=Discrete-time  UseExternalTs=off  SampleTime=-1  IntegratorMethod=Forward Euler  FilterMethod=Forward Euler  ControllerParametersSource=internal  P=1  I=1  UseKiTs=off  D=0  N=100  UseFilter=on  TunerSelectOption=Transfer Function Based (PID Tuner App)  InitialConditionSource=internal  InitialConditionForIntegrator=0  InitialConditionForFilter=0  DifferentiatorICPrevScaledInput=0  ExternalReset=none  TrackingMode=off  Kt=1  LimitOutput=off  SatLimitsSource=internal  UpperSaturationLimit=inf  LowerSaturationLimit=-inf  LinearizeAsGain=off  AntiWindupMode=none  Kb=1  POutMin=[]  POutMax=[]  IOutMin=[]  IOutMax=[]  DOutMin=[]  DOutMax=[]  NOutMin=[]  NOutMax=[]  SumOutMin=[]  SumOutMax=[]  SaturationOutMin=[]  SaturationOutMax=[]  PParamMin=[]  PParamMax=[]  IParamMin=[]  IParamMax=[]  DParamMin=[]  DParamMax=[]  NParamMin=[]  NParamMax=[]  KbParamMin=[]  KbParamMax=[]  KtParamMin=[]  KtParamMax=[]  KbOutMin=[]  KbOutMax=[]  KtOutMin=[]  KtOutMax=[]  IntegratorOutMin=[]  IntegratorOutMax=[]  FilterOutMin=[]  FilterOutMax=[]  SumI1OutMin=[]  SumI1OutMax=[]  SumI2OutMin=[]  SumI2OutMax=[]  SumI3OutMin=[]  SumI3OutMax=[]  SumI4OutMin=[]  SumI4OutMax=[]  SumDOutMin=[]  SumDOutMax=[]  DifferentiatorOutMin=[]  DifferentiatorOutMax=[]  FilterDiffOutCoefMin=[]  FilterDiffOutCoefMax=[]  ReciprocalOutMin=[]  ReciprocalOutMax=[]  SumDenOutMin=[]  SumDenOutMax=[]  SumNumOutMin=[]  SumNumOutMax=[]  DivideOutMin=[]  DivideOutMax=[]  UdiffTsProdOutMin=[]  UdiffTsProdOutMax=[]  NTsProdOutMin=[]  NTsProdOutMax=[]  UintegralTsProdOutMin=[]  UintegralTsProdOutMax=[]  UngainTsProdOutMin=[]  UngainTsProdOutMax=[]  IntegratorContinuousStateAttributes=''  IntegratorStateMustResolveToSignalObject=off  IntegratorRTWStateStorageClass=Auto  FilterContinuousStateAttributes=''  FilterStateMustResolveToSignalObject=off  FilterRTWStateStorageClass=Auto  ParallelPVariant=InternalParameters  IdealPVariant=Disabled  IVariant=InternalParameters  DVariant=InternalParameters  IntegratorVariant=Discrete  SatVariant=Disabled  AWVariant=Passthrough  PCopyVariant=Disabled  TRVariant=Disabled  FdbkBlocksVariant=Forward  IdealPFdbkVariant=Disabled  SatFdbkVariant=Disabled  DerivativeFilterVariant=ForwardEulerFilter  NVariant=InternalParameters  NCopyVariant=Disabled  FilterICVariant=InternalICsFilter  IntegratorICVariant=InternalICs  ExternalResetVariant=Disabled  TRSumVariant=Passthrough  SumFdbkVariant=Disabled  SumVariant=Sum_PID  TsampFilterVariant=InternalTs  TsampNgainVariant=Passthrough  TsampIntegralVariant=Passthrough  ExternalSaturationOutDataTypeStr=Inherit: Same as second input  aMode=0
  cfblk4 : DiscreteStateSpace  SampleTime=-1
  cfblk5 : Gain  Gain=[220768961.403727]
  cfblk6 : Constant  Value=[-135023864.093883]  SampleTime=1
  cfblk7 : Subsystem
  cfblk2 : Outport
  wires:
  cfblk6/1 -> cfblk5/1
  cfblk7/1(cfblk2) -> cfblk3/1
  cfblk5/1 -> cfblk7/1(cfblk1)
  cfblk7/2(cfblk15) -> cfblk4/1
  cfblk3/1 -> cfblk2/1

== system sampleModel1999/cfblk29/cfblk10 ==
  cfblk1 : Inport
  cfblk10 : Inport  Port=2
  cfblk11 : Inport  Port=3
  cfblk12 : Inport  Port=4
  cfblk13 : Inport  Port=5
  cfblk14 : Delay  SampleTime=1
  cfblk3 : simulink/Discrete/Transfer Fcn Lead or Lag  PoleZ=0.95  ZeroZ=0.75  ICPrevOutput=0.0  ICPrevInput=0.0  DoSatur=off
      settings: SourceProductBaseCode=SL
  cfblk4 : Reshape
  cfblk5 : Sum  Inputs=+-
  cfblk6 : Squeeze
  cfblk7 : Abs  SaturateOnIntegerOverflow=off
  cfblk8 : Constant  Value=[17011813.988466]  SampleTime=1
  cfblk9 : Constant  Value=[394036538.963661]  SampleTime=1
  cfblk2 : Outport
  wires:
  cfblk9/1 -> cfblk2/1
  cfblk11/1 -> cfblk3/1
  cfblk10/1 -> cfblk5/1
  cfblk1/1 -> cfblk5/2
  cfblk12/1 -> cfblk4/1
  cfblk6/1 -> cfblk7/1
  cfblk7/1 -> cfblk14/1
  cfblk14/1 -> cfblk6/1

== system sampleModel1999/cfblk29/cfblk11 ==
  cfblk1 : Inport
  cfblk10 : Inport  Port=2
  cfblk11 : Inport  Port=3
  cfblk3 : UnitDelay  HasFrameUpgradeWarning=on
  cfblk4 : simulink/Discrete/Transfer Fcn First Order  PoleZ=0.95  ICPrevOutput=0.0  DoSatur=off
  cfblk5 : simulink/Discrete/Transfer Fcn Real Zero  ZeroZ=0.75  ICPrevInput=0.0  DoSatur=off
      settings: SourceProductBaseCode=SL
  cfblk6 : Sqrt
  cfblk7 : Sum  Inputs=+
  cfblk8 : Abs  SaturateOnIntegerOverflow=off
  cfblk9 : ComplexToMagnitudeAngle
  cfblk2 : Outport
  wires:
  cfblk3/1 -> cfblk8/1
  cfblk8/1 -> cfblk2/1
  cfblk5/1 -> cfblk7/1
  cfblk7/1 -> cfblk4/1
  cfblk1/1 -> cfblk5/1
  cfblk10/1 -> cfblk9/1
  cfblk4/1 -> cfblk3/1
  cfblk9/1 -> cfblk6/1

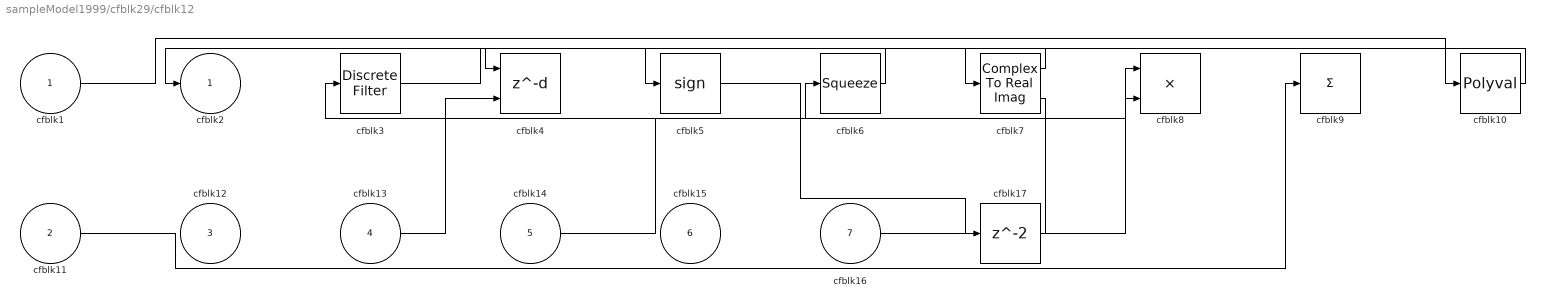
== system sampleModel1999/cfblk29/cfblk12 ==
  cfblk1 : Inport
  cfblk11 : Inport  Port=2
  cfblk12 : Inport  Port=3
  cfblk13 : Inport  Port=4
  cfblk14 : Inport  Port=5
  cfblk15 : Inport  Port=6
  cfblk16 : Inport  Port=7
  cfblk10 : Polyval  Coefs=[ +2.081618890e-019, -1.441693666e-014, +4.719686976e-010, -8.536869453e-006, +1.621573104e-001, -8.087801117e+001 ]
  cfblk17 : Delay  SampleTime=1
  cfblk3 : DiscreteFilter  SampleTime=1
  cfblk4 : Delay  DelayLengthSource=Input port  SampleTime=1
      settings: InputPortMap=u0,p1
  cfblk5 : Signum
  cfblk6 : Squeeze
  cfblk7 : ComplexToRealImag
  cfblk8 : Product
  cfblk9 : Sum  Inputs=+
  cfblk2 : Outport
  wires:
  cfblk6/1 -> cfblk2/1
  cfblk14/1 -> cfblk8/1
  cfblk7/1 -> cfblk4/1
  cfblk13/1 -> cfblk4/2
  cfblk3/1 -> cfblk5/1
  cfblk1/1 -> cfblk10/1
  cfblk10/1 -> cfblk7/1
  cfblk11/1 -> cfblk9/1
  cfblk7/2 -> cfblk6/1
  cfblk16/1 -> cfblk8/2
  cfblk5/1 -> cfblk17/1
  cfblk17/1 -> cfblk3/1

== system sampleModel1999/cfblk29/cfblk6 ==
  cfblk1 : Inport
  cfblk10 : Inport  Port=2
  cfblk11 : Inport  Port=3
  cfblk3 : UnitDelay  HasFrameUpgradeWarning=on
  cfblk4 : simulink/Discrete/Transfer Fcn Lead or Lag  PoleZ=0.95  ZeroZ=0.75  ICPrevOutput=0.0  ICPrevInput=0.0  DoSatur=off
      settings: SourceProductBaseCode=SL
  cfblk5 : simulink/Discrete/Transfer Fcn First Order  PoleZ=0.95  ICPrevOutput=0.0  DoSatur=off
  cfblk6 : PermuteDimensions
  cfblk7 : Product  Inputs=*
  cfblk8 : Constant  Value=[943506346.665642]  SampleTime=1
  cfblk9 : Constant  Value=[-757477142.227719]  SampleTime=1
  cfblk2 : Outport
  wires:
  cfblk10/1 -> cfblk7/1
  cfblk1/1 -> cfblk3/1
  cfblk9/1 -> cfblk5/1
  cfblk11/1 -> cfblk2/1
  cfblk4/1 -> cfblk6/1
  cfblk8/1 -> cfblk4/1

== system sampleModel1999/cfblk29/cfblk7 ==
  cfblk1 : Inport
  cfblk13 : Inport  Port=2
  cfblk10 : Bias  Bias=[510685833.043050]  SaturateOnIntegerOverflow=off
  cfblk11 : simulink/Math Operations/MinMax Running Resettable  Function=min  vinit=0.0
  cfblk12 : Constant  Value=[-520836228.891929]  SampleTime=1
  cfblk15 : Delay  SampleTime=1
  cfblk3 : slpidlib/PID Controller  Controller=PID  Form=Parallel  TimeDomain=Discrete-time  UseExternalTs=off  SampleTime=1  IntegratorMethod=Forward Euler  FilterMethod=Forward Euler  ControllerParametersSource=internal  P=1  I=1  UseKiTs=off  D=0  N=100  UseFilter=on  TunerSelectOption=Transfer Function Based (PID Tuner App)  InitialConditionSource=internal  InitialConditionForIntegrator=0  InitialConditionForFilter=0  DifferentiatorICPrevScaledInput=0  ExternalReset=none  TrackingMode=off  Kt=1  LimitOutput=off  SatLimitsSource=internal  UpperSaturationLimit=inf  LowerSaturationLimit=-inf  LinearizeAsGain=off  AntiWindupMode=none  Kb=1  POutMin=[]  POutMax=[]  IOutMin=[]  IOutMax=[]  DOutMin=[]  DOutMax=[]  NOutMin=[]  NOutMax=[]  SumOutMin=[]  SumOutMax=[]  SaturationOutMin=[]  SaturationOutMax=[]  PParamMin=[]  PParamMax=[]  IParamMin=[]  IParamMax=[]  DParamMin=[]  DParamMax=[]  NParamMin=[]  NParamMax=[]  KbParamMin=[]  KbParamMax=[]  KtParamMin=[]  KtParamMax=[]  KbOutMin=[]  KbOutMax=[]  KtOutMin=[]  KtOutMax=[]  IntegratorOutMin=[]  IntegratorOutMax=[]  FilterOutMin=[]  FilterOutMax=[]  SumI1OutMin=[]  SumI1OutMax=[]  SumI2OutMin=[]  SumI2OutMax=[]  SumI3OutMin=[]  SumI3OutMax=[]  SumI4OutMin=[]  SumI4OutMax=[]  SumDOutMin=[]  SumDOutMax=[]  DifferentiatorOutMin=[]  DifferentiatorOutMax=[]  FilterDiffOutCoefMin=[]  FilterDiffOutCoefMax=[]  ReciprocalOutMin=[]  ReciprocalOutMax=[]  SumDenOutMin=[]  SumDenOutMax=[]  SumNumOutMin=[]  SumNumOutMax=[]  DivideOutMin=[]  DivideOutMax=[]  UdiffTsProdOutMin=[]  UdiffTsProdOutMax=[]  NTsProdOutMin=[]  NTsProdOutMax=[]  UintegralTsProdOutMin=[]  UintegralTsProdOutMax=[]  UngainTsProdOutMin=[]  UngainTsProdOutMax=[]  IntegratorContinuousStateAttributes=''  IntegratorStateMustResolveToSignalObject=off  IntegratorRTWStateStorageClass=Auto  FilterContinuousStateAttributes=''  FilterStateMustResolveToSignalObject=off  FilterRTWStateStorageClass=Auto  ParallelPVariant=InternalParameters  IdealPVariant=Disabled  IVariant=InternalParameters  DVariant=InternalParameters  IntegratorVariant=Discrete  SatVariant=Disabled  AWVariant=Passthrough  PCopyVariant=Disabled  TRVariant=Disabled  FdbkBlocksVariant=Forward  IdealPFdbkVariant=Disabled  SatFdbkVariant=Disabled  DerivativeFilterVariant=ForwardEulerFilter  NVariant=InternalParameters  NCopyVariant=Disabled  FilterICVariant=InternalICsFilter  IntegratorICVariant=InternalICs  ExternalResetVariant=Disabled  TRSumVariant=Passthrough  SumFdbkVariant=Disabled  SumVariant=Sum_PID  TsampFilterVariant=InternalTs  TsampNgainVariant=Passthrough  TsampIntegralVariant=Passthrough  ExternalSaturationOutDataTypeStr=Inherit: Same as second input  aMode=0
  cfblk4 : DiscreteTransferFcn  SampleTime=1
  cfblk5 : DiscreteFilter  SampleTime=1
  cfblk6 : slpidlib/PID Controller (2DOF)  Controller=PID  Form=Parallel  TimeDomain=Discrete-time  UseExternalTs=off  SampleTime=1  IntegratorMethod=Forward Euler  FilterMethod=Forward Euler  ControllerParametersSource=internal  P=1  I=1  UseKiTs=off  D=0  N=100  UseFilter=on  b=1  c=1  TunerSelectOption=Transfer Function Based (PID Tuner App)  InitialConditionSource=internal  InitialConditionForIntegrator=0  InitialConditionForFilter=0  DifferentiatorICPrevScaledInput=0  ExternalReset=none  TrackingMode=off  Kt=1  LimitOutput=off  SatLimitsSource=internal  UpperSaturationLimit=inf  LowerSaturationLimit=-inf  LinearizeAsGain=off  AntiWindupMode=none  Kb=1  POutMin=[]  POutMax=[]  IOutMin=[]  IOutMax=[]  DOutMin=[]  DOutMax=[]  NOutMin=[]  NOutMax=[]  bOutMin=[]  bOutMax=[]  cOutMin=[]  cOutMax=[]  SumOutMin=[]  SumOutMax=[]  SaturationOutMin=[]  SaturationOutMax=[]  PParamMin=[]  PParamMax=[]  IParamMin=[]  IParamMax=[]  DParamMin=[]  DParamMax=[]  NParamMin=[]  NParamMax=[]  bParamMin=[]  bParamMax=[]  cParamMin=[]  cParamMax=[]  KbParamMin=[]  KbParamMax=[]  KtParamMin=[]  KtParamMax=[]  KbOutMin=[]  KbOutMax=[]  KtOutMin=[]  KtOutMax=[]  IntegratorOutMin=[]  IntegratorOutMax=[]  FilterOutMin=[]  FilterOutMax=[]  SumI1OutMin=[]  SumI1OutMax=[]  SumI2OutMin=[]  SumI2OutMax=[]  SumI3OutMin=[]  SumI3OutMax=[]  SumI4OutMin=[]  SumI4OutMax=[]  SumDOutMin=[]  SumDOutMax=[]  Sum1OutMin=[]  Sum1OutMax=[]  Sum2OutMin=[]  Sum2OutMax=[]  Sum3OutMin=[]  Sum3OutMax=[]  DifferentiatorOutMin=[]  DifferentiatorOutMax=[]  FilterDiffOutCoefMin=[]  FilterDiffOutCoefMax=[]  ReciprocalOutMin=[]  ReciprocalOutMax=[]  SumDenOutMin=[]  SumDenOutMax=[]  SumNumOutMin=[]  SumNumOutMax=[]  DivideOutMin=[]  DivideOutMax=[]  UdiffTsProdOutMin=[]  UdiffTsProdOutMax=[]  NTsProdOutMin=[]  NTsProdOutMax=[]  UintegralTsProdOutMin=[]  UintegralTsProdOutMax=[]  UngainTsProdOutMin=[]  UngainTsProdOutMax=[]  IntegratorContinuousStateAttributes=''  IntegratorStateMustResolveToSignalObject=off  IntegratorRTWStateStorageClass=Auto  FilterContinuousStateAttributes=''  FilterStateMustResolveToSignalObject=off  FilterRTWStateStorageClass=Auto  ParallelPVariant=InternalParameters  IdealPVariant=Disabled  IVariant=InternalParameters  DVariant=InternalParameters  bVariant=InternalParameters  cVariant=InternalParameters  IntegratorVariant=Discrete  SatVariant=Disabled  AWVariant=Passthrough  PCopyVariant=Disabled  TRVariant=Disabled  FdbkBlocksVariant=Forward  IdealPFdbkVariant=Disabled  SatFdbkVariant=Disabled  DerivativeFilterVariant=ForwardEulerFilter  NVariant=InternalParameters  NCopyVariant=Disabled  FilterICVariant=InternalICsFilter  IntegratorICVariant=InternalICs  ExternalResetVariant=Disabled  TRSumVariant=Passthrough  SumFdbkVariant=Disabled  SumVariant=Sum_PID  TsampFilterVariant=InternalTs  TsampNgainVariant=Passthrough  TsampIntegralVariant=Passthrough  ExternalSaturationOutDataTypeStr=Inherit: Same as second input
      settings: SourceProductBaseCode=SL
  cfblk7 : DiscreteZeroPole  Poles=[0 0.5]  Gain=1
  cfblk8 : Reshape
  cfblk9 : MinMax  Inputs=2
  cfblk2 : Outport
  cfblk14 : Outport  Port=2
  wires:
  cfblk9/1 -> cfblk14/1, cfblk5/1
  cfblk1/1 -> cfblk6/1
  cfblk7/1 -> cfblk4/1, cfblk11/2
  cfblk3/1 -> cfblk8/1
  cfblk4/1 -> cfblk11/1
  cfblk6/1 -> cfblk9/1
  cfblk12/1 -> cfblk2/1
  cfblk11/1 -> cfblk3/1
  cfblk13/1 -> cfblk10/1
  cfblk5/1 -> cfblk7/1
  cfblk10/1 -> cfblk6/2
  cfblk8/1 -> cfblk15/1
  cfblk15/1 -> cfblk9/2

== system sampleModel1999/cfblk29/cfblk8 ==
  cfblk1 : Inport
  cfblk10 : Inport  Port=2
  cfblk11 : Inport  Port=3
  cfblk12 : Inport  Port=4
  cfblk13 : Delay  SampleTime=1
  cfblk3 : Sum  Inputs=+-
  cfblk4 : Sum  Inputs=+-
  cfblk5 : Sum  Inputs=+
  cfblk6 : Sum
  cfblk7 : Abs  SaturateOnIntegerOverflow=off
  cfblk8 : Assignment  DiagnosticForDimensions=Warning  IndexOptions=Index vector (dialog)  Indices=1  OutputSizes=1
  cfblk9 : Constant  Value=[732039654.390262]  SampleTime=1
  cfblk2 : Outport
  wires:
  cfblk12/1 -> cfblk2/1
  cfblk11/1 -> cfblk8/1
  cfblk1/1 -> cfblk7/1
  cfblk7/1 -> cfblk4/1
  cfblk6/1 -> cfblk3/1
  cfblk5/1 -> cfblk8/2
  cfblk9/1 -> cfblk5/1
  cfblk10/1 -> cfblk3/2
  cfblk8/1 -> cfblk6/1
  cfblk4/1 -> cfblk6/2
  cfblk3/1 -> cfblk13/1
  cfblk13/1 -> cfblk4/2

== system sampleModel1999/cfblk29/cfblk9 ==
  cfblk1 : Inport
  cfblk7 : Inport  Port=2
  cfblk3 : Delay  SampleTime=1
  cfblk4 : simulink/Math Operations/Slider Gain  gain=1  low=0  high=2
  cfblk5 : Sum  Inputs=+
  cfblk6 : UnaryMinus
  cfblk2 : Outport
  cfblk8 : Outport  Port=2
  wires:
  cfblk1/1 -> cfblk4/1
  cfblk5/1 -> cfblk3/1
  cfblk3/1 -> cfblk6/1
  cfblk6/1 -> cfblk2/1
  cfblk7/1 -> cfblk5/1
  cfblk4/1 -> cfblk8/1

== system sampleModel1999/cfblk30/cfblk10 ==
  cfblk1 : Inport
  cfblk12 : Inport  Port=2
  cfblk13 : Inport  Port=3
  cfblk14 : Inport  Port=4
  cfblk15 : Inport  Port=5
  cfblk16 : Inport  Port=6
  cfblk10 : simulink/Math Operations/Slider Gain  gain=1  low=0  high=2
  cfblk11 : Sqrt  Operator=rSqrt  AlgorithmType=Newton-Raphson
  cfblk3 : Delay  SampleTime=1
  cfblk4 : Signum
  cfblk5 : Sqrt
  cfblk6 : Sum  Inputs=+-
  cfblk7 : DotProduct  OutDataTypeStr=Inherit: Inherit via internal rule
  cfblk8 : Math  Operator=magnitude^2
  cfblk9 : Sqrt
  cfblk2 : Outport
  cfblk17 : Outport  Port=2
  wires:
  cfblk9/1 -> cfblk8/1
  cfblk13/1 -> cfblk7/1
  cfblk6/1 -> cfblk2/1
  cfblk11/1 -> cfblk3/1
  cfblk14/1 -> cfblk11/1
  cfblk16/1 -> cfblk9/1
  cfblk15/1 -> cfblk10/1
  cfblk10/1 -> cfblk17/1
  cfblk3/1 -> cfblk5/1
  cfblk5/1 -> cfblk6/1
  cfblk1/1 -> cfblk7/2
  cfblk12/1 -> cfblk4/1
  cfblk8/1 -> cfblk6/2
